simulink model "Tugas_no_1"  (R2022b)
settings: Solver=VariableStepAuto  StartTime=0.0  StopTime=10.0  RelTol=1e-3
settings Model: Creator=hp  LastModifiedBy=hp

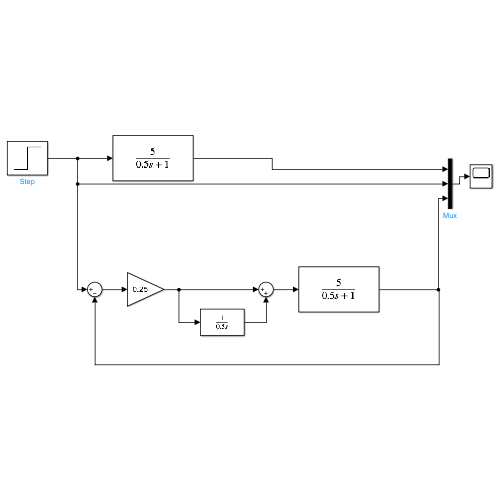
[thumbnail: Simulink's stored preview of the top-level diagram]
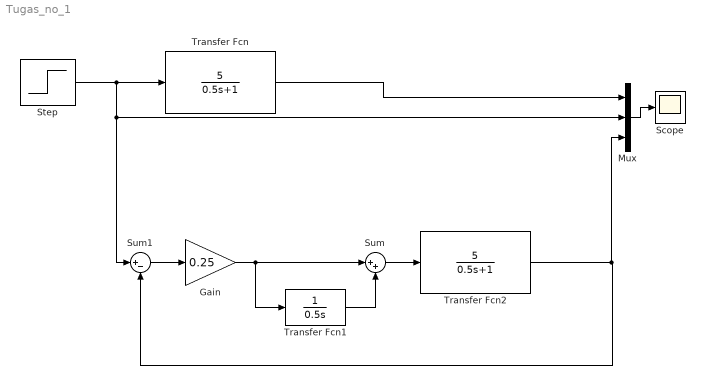
== system Tugas_no_1 ==
  Gain : Gain  Gain=0.25
  Mux : Mux  Inputs=3
  Scope : Scope
  Step : Step  SampleTime=0
  Sum : Sum  Inputs=|++
  Sum1 : Sum  Inputs=|+-
  Transfer Fcn : TransferFcn  Numerator=[5]  Denominator=[0.5 1]
  Transfer Fcn1 : TransferFcn  Denominator=[0.5 0]
  Transfer Fcn2 : TransferFcn  Numerator=[5]  Denominator=[0.5 1]
  wires:
  Step/1 -> Sum1/1, Mux/2, Transfer Fcn/1
  Transfer Fcn/1 -> Mux/1
  Mux/1 -> Scope/1
  Gain/1 -> Transfer Fcn1/1, Sum/1
  Transfer Fcn1/1 -> Sum/2
  Sum/1 -> Transfer Fcn2/1
  Sum1/1 -> Gain/1
  Transfer Fcn2/1 -> Mux/3, Sum1/2
